simulink model "Cont_fullstate"  (R2020a)
settings: Solver=ode45  StartTime=0.0  StopTime=20  RelTol=1e-5
values from neighbouring files (symbols this model uses):
  A = [   0       1               0           0 ... (first row only)    [main_code.m]
  Ad = sys_d.a    [main_code.m]
  B = [   0 ... (first row only)    [main_code.m]
  b = 0.5    [main_code.m]
  Bd = sys_d.b    [main_code.m]
  C = [1   0   0   0 ... (first row only)    [main_code.m]
  Cd = sys_d.c    [main_code.m]
  Current_saturation = 2000    [main_code.m]
  D = [0 ... (first row only)    [main_code.m]
  Dd = sys_d.d    [main_code.m]
  g = 9.8    [main_code.m]
  I = (m*l^2)/3    (= 0.002646)    [main_code.m]
  K = lqr(A,B,Q,R)    [main_code.m]
  Kd = dlqr(Ad,Bd,Q,R)    [main_code.m]
  l = 0.21    [main_code.m]
  L = place(A',C',P)'    [main_code.m]
  Ld = place(Ad',Cd',Pd)'    [main_code.m]
  m = 0.18    [main_code.m]
  M = 0.195    [main_code.m]
  N_to_mAmp = 260    [main_code.m]
  Nc = 1/dcgain(sys_cl(1))    [main_code.m]
  Ndc = 1/dcgain(sys_d_cl(1))    [main_code.m]
  Ts = 1/100    (= 0.01)    [main_code.m]
  X0 = [0 0 pi 0.1]'    [main_code.m]
undefined symbols (not defined in the file or in its folder): X, Y, Z
libraries: sm_lib x8, nesl_utility x6
settings Model: Creator=imkis  LastModifiedBy=imkis
settings SolverCC: AlgebraicLoopSolver=LineSearch

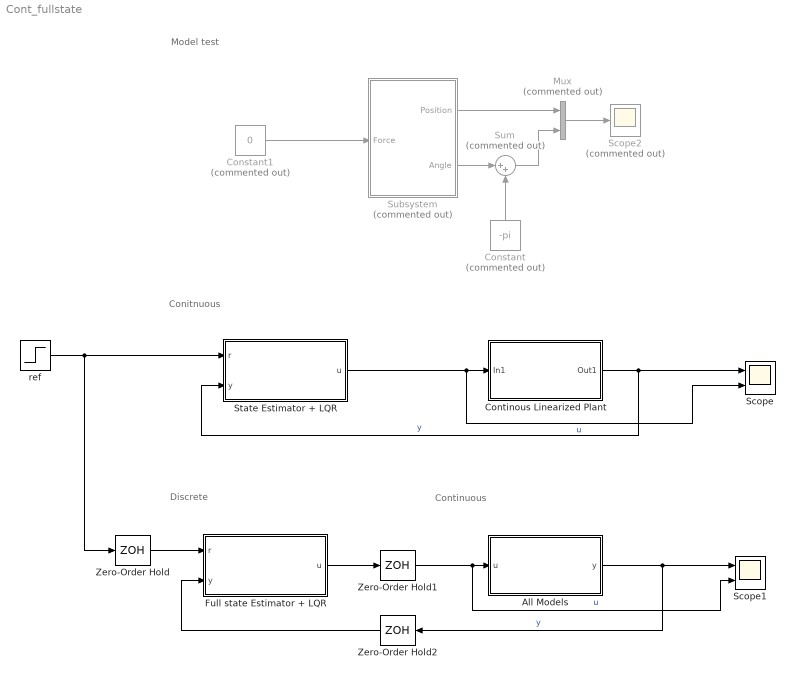
== system Cont_fullstate ==
  note: Model test
  note: Conitnuous
  note: Continuous
  note: Discrete
  All Models : Subsystem
  Constant : Constant  Commented=on  Value=-pi
  Constant1 : Constant  Commented=on  Value=0
  Continous Linearized Plant : Subsystem
  "Full state Estimator + LQR " : Subsystem
  Mux : Mux  Commented=on  Inputs=2
  Scope : Scope  NumInputPorts=2
  Scope1 : Scope  NumInputPorts=2
  Scope2 : Scope  Commented=on
  "State Estimator + LQR " : Subsystem
  Subsystem : Subsystem  Commented=on
  Sum : Sum  Commented=on  Inputs=|++
  Zero-Order Hold : ZeroOrderHold  SampleTime=Ts
  Zero-Order Hold1 : ZeroOrderHold  SampleTime=Ts
  Zero-Order Hold2 : ZeroOrderHold  SampleTime=Ts
  ref : Step  After=0.1  SampleTime=0
  wires:
  Continous Linearized Plant/1(Out1) -> Scope/1, "State Estimator + LQR "/2(y)  "y"
  "State Estimator + LQR "/1(u) -> Scope/2, Continous Linearized Plant/1(In1)  "u"
  ref/1 -> Zero-Order Hold/1, "State Estimator + LQR "/1(r)
  Zero-Order Hold/1 -> "Full state Estimator + LQR "/1(r)
  "Full state Estimator + LQR "/1(u) -> Zero-Order Hold1/1
  All Models/1(y) -> Scope1/1, Zero-Order Hold2/1  "y"
  Zero-Order Hold1/1 -> Scope1/2, All Models/1(u)  "u"
  Zero-Order Hold2/1 -> "Full state Estimator + LQR "/2(y)
  Subsystem/2(Angle) -> Sum/1
  Mux/1 -> Scope2/1
  Constant1/1 -> Subsystem/1(Force)
  Sum/1 -> Mux/2
  Subsystem/1(Position) -> Mux/1
  Constant/1 -> Sum/2

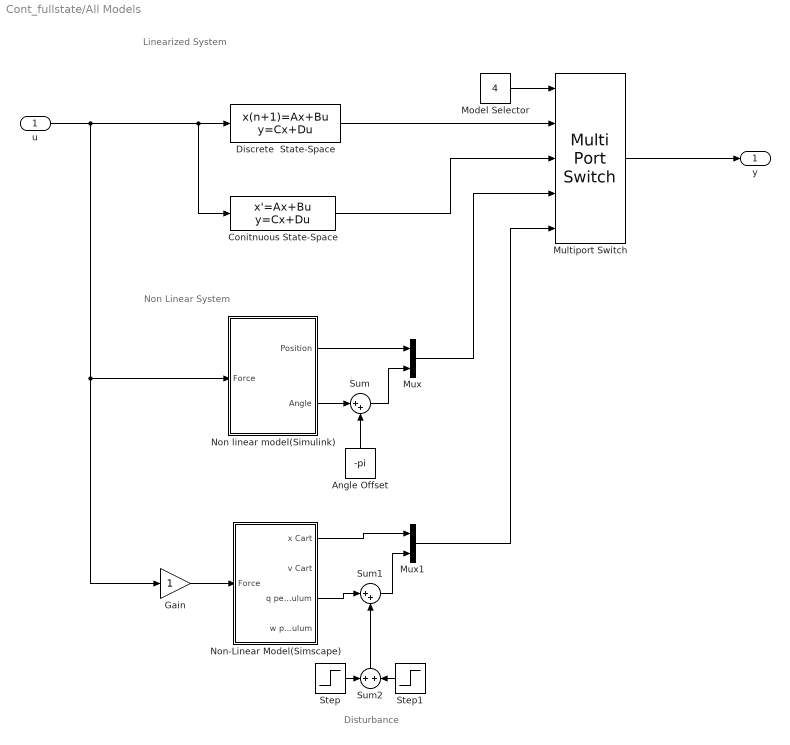
== system Cont_fullstate/All Models ==
  note: Disturbance
  note: Non Linear System
  note: Linearized System
  u : Inport
  Angle Offset : Constant  Value=-pi
  Conitnuous State-Space : StateSpace  A=A  B=B  C=C  D=D  InitialCondition=X0
  Discrete  State-Space : DiscreteStateSpace  A=Ad  B=Bd  C=Cd  D=Dd  InitialCondition=X0  SampleTime=Ts
  Gain : Gain
  Model Selector : Constant  Value=4
  Multiport Switch : MultiPortSwitch  Inputs=4
  Mux : Mux  Inputs=2
  Mux1 : Mux  Inputs=2
  "Non linear model(Simulink) " : Subsystem
  Non-Linear Model(Simscape) : Subsystem
  Step : Step  Time=5  After=0.1  SampleTime=0
  Step1 : Step  Time=5.05  After=-0.1  SampleTime=0
  Sum : Sum  Inputs=|++
  Sum1 : Sum  Inputs=|++
  Sum2 : Sum  Inputs=+|+
  y : Outport
  wires:
  Discrete  State-Space/1 -> Multiport Switch/2
  Conitnuous State-Space/1 -> Multiport Switch/3
  Multiport Switch/1 -> y/1
  "Non linear model(Simulink) "/2(Angle) -> Sum/1
  u/1 -> Conitnuous State-Space/1, Discrete  State-Space/1, "Non linear model(Simulink) "/1(Force), Gain/1
  Sum/1 -> Mux/2
  "Non linear model(Simulink) "/1(Position) -> Mux/1
  Angle Offset/1 -> Sum/2
  Sum1/1 -> Mux1/2
  Non-Linear Model(Simscape)/3(q pendulum) -> Sum1/1
  Non-Linear Model(Simscape)/1(x Cart) -> Mux1/1
  Mux1/1 -> Multiport Switch/5
  Mux/1 -> Multiport Switch/4
  Model Selector/1 -> Multiport Switch/1
  Gain/1 -> Non-Linear Model(Simscape)/1(Force)
  Step/1 -> Sum2/1
  Step1/1 -> Sum2/2
  Sum2/1 -> Sum1/2

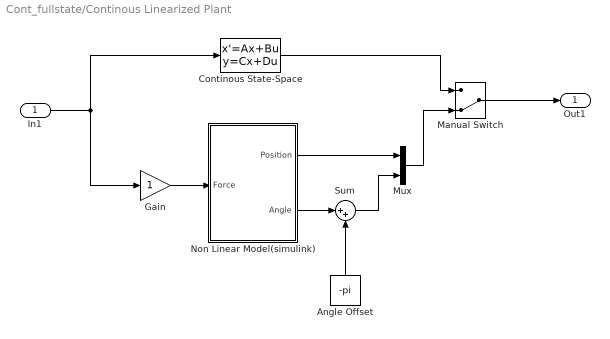
== system Cont_fullstate/Continous Linearized Plant ==
  In1 : Inport
  Angle Offset : Constant  Value=-pi
  Continous State-Space : StateSpace  A=A  B=B  C=C  D=D  InitialCondition=X0
  Gain : Gain
  Manual Switch : ManualSwitch  CurrentSetting=0
  Mux : Mux  Inputs=2
  Non Linear Model(simulink) : Subsystem
  Sum : Sum  Inputs=|++
  Out1 : Outport
  wires:
  Continous State-Space/1 -> Manual Switch/1
  Gain/1 -> Non Linear Model(simulink)/1(Force)
  Mux/1 -> Manual Switch/2
  Manual Switch/1 -> Out1/1
  Non Linear Model(simulink)/2(Angle) -> Sum/1
  Sum/1 -> Mux/2
  Non Linear Model(simulink)/1(Position) -> Mux/1
  Angle Offset/1 -> Sum/2
  In1/1 -> Continous State-Space/1, Gain/1

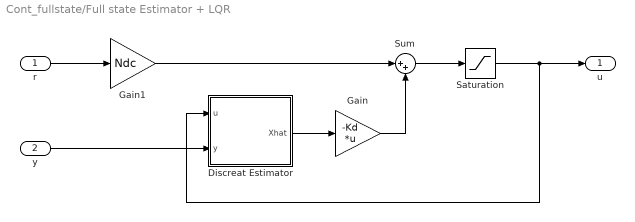
== system Cont_fullstate/Full state Estimator + LQR  ==
  r : Inport
  y : Inport  Port=2
  Discreat Estimator : Subsystem
  Gain : Gain  Gain=-Kd  Multiplication=Matrix(K*u)
  Gain1 : Gain  Gain=Ndc
  Saturation : Saturate  UpperLimit=Current_saturation/N_to_mAmp  LowerLimit=-Current_saturation/N_to_mAmp
  Sum : Sum  Inputs=|++
  u : Outport
  wires:
  Gain1/1 -> Sum/1
  Sum/1 -> Saturation/1
  y/1 -> Discreat Estimator/2(y)
  Discreat Estimator/1(Xhat) -> Gain/1
  Gain/1 -> Sum/2
  r/1 -> Gain1/1
  Saturation/1 -> u/1, Discreat Estimator/1(u)

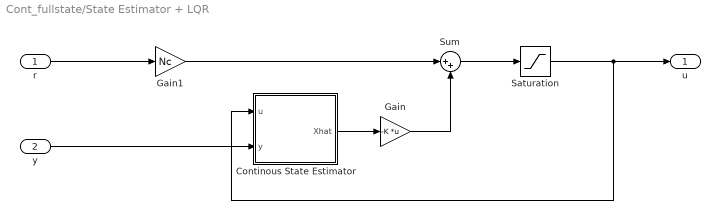
== system Cont_fullstate/State Estimator + LQR  ==
  r : Inport
  y : Inport  Port=2
  Continous State Estimator : Subsystem
  Gain : Gain  Gain=-K  Multiplication=Matrix(K*u)
  Gain1 : Gain  Gain=Nc
  Saturation : Saturate  UpperLimit=8  LowerLimit=-8
  Sum : Sum  Inputs=|++
  u : Outport
  wires:
  Gain1/1 -> Sum/1
  Sum/1 -> Saturation/1
  y/1 -> Continous State Estimator/2(y)
  Continous State Estimator/1(Xhat) -> Gain/1
  Gain/1 -> Sum/2
  r/1 -> Gain1/1
  Saturation/1 -> Continous State Estimator/1(u), u/1

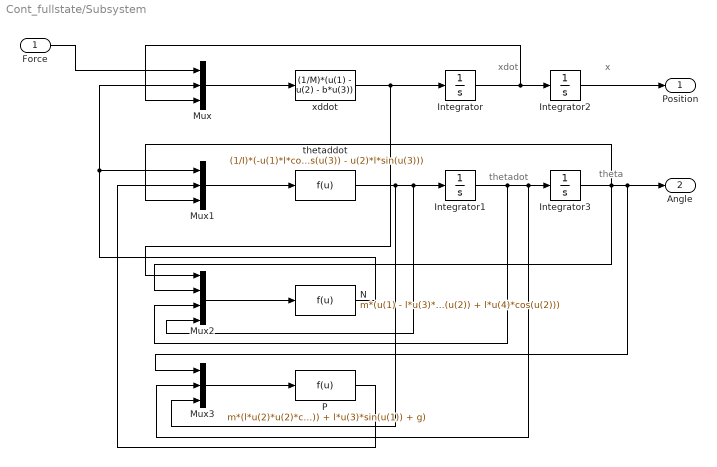
== system Cont_fullstate/Subsystem ==
  note: theta
  note: x
  note: thetadot
  note: xdot
  Force : Inport
  Integrator : Integrator  InitialCondition=X0(2)  ContinuousStateAttributes='xdot'
  Integrator1 : Integrator  InitialCondition=X0(4)  ContinuousStateAttributes='thetadot'
  Integrator2 : Integrator  InitialCondition=X0(1)  ContinuousStateAttributes='x'
  Integrator3 : Integrator  InitialCondition=X0(3)  ContinuousStateAttributes='theta'
  Mux : Mux  Inputs=3
  Mux1 : Mux  Inputs=3
  Mux2 : Mux
  Mux3 : Mux  Inputs=3
  N : Fcn  Expr=m*(u(1) - l*u(3)*u(3)*sin(u(2)) + l*u(4)*cos(u(2)))
  P : Fcn  Expr=m*(l*u(2)*u(2)*cos(u(1)) + l*u(3)*sin(u(1)) + g)
  thetaddot : Fcn  Expr=(1/I)*(-u(1)*l*cos(u(3)) - u(2)*l*sin(u(3)))
  xddot : Fcn  Expr=(1/M)*(u(1) - u(2) - b*u(3))
  Position : Outport
  Angle : Outport  Port=2
  wires:
  Force/1 -> Mux/1
  Mux2/1 -> N/1
  Mux/1 -> xddot/1
  P/1 -> Mux1/2
  Mux3/1 -> P/1
  N/1 -> Mux1/1, Mux/2
  Mux1/1 -> thetaddot/1
  xddot/1 -> Mux2/1, Integrator/1
  Integrator2/1 -> Position/1
  thetaddot/1 -> Mux3/3, Mux2/4, Integrator1/1
  Integrator/1 -> Mux/3, Integrator2/1
  Integrator1/1 -> Mux2/3, Mux3/2, Integrator3/1
  Integrator3/1 -> Mux2/2, Mux1/3, Angle/1, Mux3/1

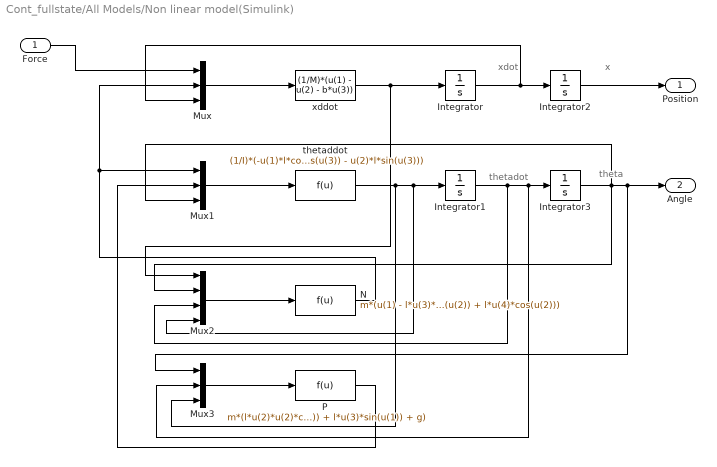
== system Cont_fullstate/All Models/Non linear model(Simulink)  ==
  note: theta
  note: x
  note: thetadot
  note: xdot
  Force : Inport
  Integrator : Integrator  ContinuousStateAttributes='xdot'
  Integrator1 : Integrator  ContinuousStateAttributes='thetadot'
  Integrator2 : Integrator  ContinuousStateAttributes='x'
  Integrator3 : Integrator  InitialCondition=pi  ContinuousStateAttributes='theta'
  Mux : Mux  Inputs=3
  Mux1 : Mux  Inputs=3
  Mux2 : Mux
  Mux3 : Mux  Inputs=3
  N : Fcn  Expr=m*(u(1) - l*u(3)*u(3)*sin(u(2)) + l*u(4)*cos(u(2)))
  P : Fcn  Expr=m*(l*u(2)*u(2)*cos(u(1)) + l*u(3)*sin(u(1)) + g)
  thetaddot : Fcn  Expr=(1/I)*(-u(1)*l*cos(u(3)) - u(2)*l*sin(u(3)))
  xddot : Fcn  Expr=(1/M)*(u(1) - u(2) - b*u(3))
  Position : Outport
  Angle : Outport  Port=2
  wires:
  Force/1 -> Mux/1
  Mux2/1 -> N/1
  Mux/1 -> xddot/1
  P/1 -> Mux1/2
  Mux3/1 -> P/1
  N/1 -> Mux1/1, Mux/2
  Mux1/1 -> thetaddot/1
  xddot/1 -> Mux2/1, Integrator/1
  Integrator2/1 -> Position/1
  thetaddot/1 -> Mux3/3, Mux2/4, Integrator1/1
  Integrator/1 -> Mux/3, Integrator2/1
  Integrator1/1 -> Mux2/3, Mux3/2, Integrator3/1
  Integrator3/1 -> Mux2/2, Mux1/3, Angle/1, Mux3/1

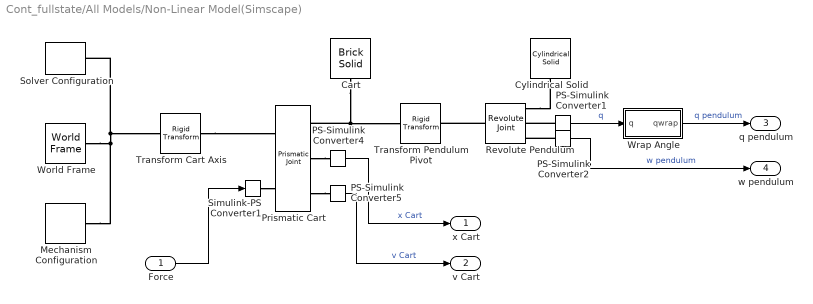
== system Cont_fullstate/All Models/Non-Linear Model(Simscape) ==
  Force : Inport
  Cart : sm_lib/Body Elements/Brick Solid  GraphicAmbientColor=[0.15 0.15 0.15 1.0]  BasedOnType=Density  BrickDimensions=[0.05 0.05 0.05]  BrickDimensionUnits=m  CenterOfMass=[0 0 0]  CenterOfMassUnits=m  GraphicDiffuseColor=[0.8 0.45 0]  Density=1000  DensityUnits=kg/m^3  DoExposeReferenceFrame=on  GraphicEmissiveColor=[0.0 0.0 0.0 1.0]  ExportEntireGeometry=off  SerializedFrames=<Frames/>  MarkerShape=Sphere  MarkerSize=10  GraphicType=FromGeometry  InertiaType=PointMass  Mass=M  MassUnits=kg  MomentsOfInertia=[1 1 1]  MomentsOfInertiaUnits=kg*m^2  GraphicOpacity=1.0  ProductsOfInertia=[0 0 0]  ProductsOfInertiaUnits=kg*m^2  GraphicShininess=75  GraphicSpecularColor=[0.5 0.5 0.5 1.0]  GraphicVisPropType=SimpleVisualProperties
  Cylindrical Solid : sm_lib/Body Elements/Cylindrical Solid  GraphicAmbientColor=[0.15 0.15 0.15 1.0]  BasedOnType=Mass  CenterOfMass=[0 0 0]  CenterOfMassUnits=m  GraphicDiffuseColor=[0.5 0.5 0.5]  CylinderLength=l*2  CylinderLengthUnits=m  CylinderRadius=0.004  CylinderRadiusUnits=m  Density=1000  DensityUnits=kg/m^3  DoExposeReferenceFrame=off  GraphicEmissiveColor=[0.0 0.0 0.0 1.0]  ExportEntireGeometry=off  SerializedFrames=<Frames><Frame><Id>Frame1</Id><Value><Name>B</Name><Origin><Source>GeometricFeature</Source><FeatureName>bottom curve</FeatureName></Origin><PrimaryAxis><DefinedDirection>-X</DefinedDirection><Source>ReferenceFrame</Source><SourceDirection>+Z</SourceDirection><FeatureName></FeatureName></PrimaryAxis><SecondaryAxis><DefinedDirection>+Y</DefinedDirection><Source>ReferenceFrame</Source><SourceDirection>+X</SourceDirection><FeatureName></FeatureName></SecondaryAxis></Value></Frame></Frames>  MarkerShape=Sphere  MarkerSize=10  GraphicType=FromGeometry  InertiaType=CalculateFromGeometry  Mass=m  MassUnits=kg  MomentsOfInertia=[1 1 1]  MomentsOfInertiaUnits=kg*m^2  GraphicOpacity=1.0  ProductsOfInertia=[0 0 0]  ProductsOfInertiaUnits=kg*m^2  GraphicShininess=75  GraphicSpecularColor=[0.5 0.5 0.5 1.0]  GraphicVisPropType=SimpleVisualProperties
  Mechanism Configuration : sm_lib/Utilities/Mechanism Configuration  UniformGravity=Constant  GravityVector=[0 0 -9.80665]  GravityUnits=m/s^2  LinearizationDelta=0.001
  PS-Simulink Converter1 : nesl_utility/PS-Simulink Converter  PhysicalDomain=network_engine_domain  SubClassName=ps_output  LeftPortType=input  RightPortType=output  PseudoPeriodic=off  Frequencies=[]  Unit=rad  AffineConversion=off
  PS-Simulink Converter2 : nesl_utility/PS-Simulink Converter  PhysicalDomain=network_engine_domain  SubClassName=ps_output  LeftPortType=input  RightPortType=output  PseudoPeriodic=off  Frequencies=[]  Unit=rad/s  AffineConversion=off
  PS-Simulink Converter4 : nesl_utility/PS-Simulink Converter  PhysicalDomain=network_engine_domain  SubClassName=ps_output  LeftPortType=input  RightPortType=output  PseudoPeriodic=off  Frequencies=[]  Unit=m  AffineConversion=off
  PS-Simulink Converter5 : nesl_utility/PS-Simulink Converter  PhysicalDomain=network_engine_domain  SubClassName=ps_output  LeftPortType=input  RightPortType=output  PseudoPeriodic=off  Frequencies=[]  Unit=m/s  AffineConversion=off
  Prismatic Cart : sm_lib/Joints/Prismatic Joint  JointMode=Normal  SenseConstraintForce=off  SenseConstraintForceX=off  SenseConstraintForceY=off  SenseConstraintForceZ=off  SenseConstraintTorque=off  SenseConstraintTorqueX=off  SenseConstraintTorqueY=off  SenseConstraintTorqueZ=off  SenseTotalForce=off  SenseTotalForceX=off  SenseTotalForceY=off  SenseTotalForceZ=off  SenseTotalTorque=off  SenseTotalTorqueX=off  SenseTotalTorqueY=off  SenseTotalTorqueZ=off  CompositeWrenchDir=FollowerOnBase  CompositeWrenchFrame=BaseFrame  EquilibriumPosition=0  EquilibriumPositionUnits=m  SpringStiffness=0  SpringStiffnessUnits=N/m  DampingCoefficient=b  DampingCoefficientUnits=N/(m/s)  TorqueActuationMode=InputTorque  MotionActuationMode=ComputedMotion  SensePosition=on  SenseVelocity=on  SenseAcceleration=off  SenseTorqueForce=off  SenseLowerLimitTorqueForce=off  SenseUpperLimitTorqueForce=off  LowerLimitSpecify=on  LowerLimitBound=-0.2  LowerLimitBoundUnits=m  LowerLimitStiffness=1e6  LowerLimitStiffnessUnits=N/m  LowerLimitDamping=1e3  LowerLimitDampingUnits=N/(m/s)  LowerLimitTransitionRegionWidth=1e-4  LowerLimitTransitionRegionWidthUnits=m  UpperLimitSpecify=on  UpperLimitBound=0.2  UpperLimitBoundUnits=m  UpperLimitStiffness=1e6  UpperLimitStiffnessUnits=N/m  UpperLimitDamping=1e3  UpperLimitDampingUnits=N/(m/s)  UpperLimitTransitionRegionWidth=1e-4  UpperLimitTransitionRegionWidthUnits=m  PositionTargetSpecify=off  PositionTargetPriority=High  PositionTargetValue=0  PositionTargetValueUnits=m  VelocityTargetSpecify=off  VelocityTargetPriority=High  VelocityTargetValue=0  VelocityTargetValueUnits=m/s
  Revolute Pendulum : sm_lib/Joints/Revolute Joint  JointMode=Normal  SenseConstraintForce=off  SenseConstraintForceX=off  SenseConstraintForceY=off  SenseConstraintForceZ=off  SenseConstraintTorque=off  SenseConstraintTorqueX=off  SenseConstraintTorqueY=off  SenseConstraintTorqueZ=off  SenseTotalForce=off  SenseTotalForceX=off  SenseTotalForceY=off  SenseTotalForceZ=off  SenseTotalTorque=off  SenseTotalTorqueX=off  SenseTotalTorqueY=off  SenseTotalTorqueZ=off  CompositeWrenchDir=FollowerOnBase  CompositeWrenchFrame=BaseFrame  EquilibriumPosition=0  EquilibriumPositionUnits=deg  SpringStiffness=0  SpringStiffnessUnits=N*m/deg  DampingCoefficient=0  DampingCoefficientUnits=N*m/(deg/s)  TorqueActuationMode=NoTorque  MotionActuationMode=ComputedMotion  SensePosition=on  SenseVelocity=on  SenseAcceleration=off  SenseTorqueForce=off  SenseLowerLimitTorqueForce=off  SenseUpperLimitTorqueForce=off  LowerLimitSpecify=off  LowerLimitBound=-90  LowerLimitBoundUnits=deg  LowerLimitStiffness=1e4  LowerLimitStiffnessUnits=N*m/deg  LowerLimitDamping=10  LowerLimitDampingUnits=N*m/(deg/s)  LowerLimitTransitionRegionWidth=0.1  LowerLimitTransitionRegionWidthUnits=deg  UpperLimitSpecify=off  UpperLimitBound=90  UpperLimitBoundUnits=deg  UpperLimitStiffness=1e4  UpperLimitStiffnessUnits=N*m/deg  UpperLimitDamping=10  UpperLimitDampingUnits=N*m/(deg/s)  UpperLimitTransitionRegionWidth=0.1  UpperLimitTransitionRegionWidthUnits=deg  PositionTargetSpecify=off  PositionTargetPriority=High  PositionTargetValue=0  PositionTargetValueUnits=deg  VelocityTargetSpecify=off  VelocityTargetPriority=High  VelocityTargetValue=0  VelocityTargetValueUnits=deg/s
  Simulink-PS Converter1 : nesl_utility/Simulink-PS Converter  PhysicalDomain=network_engine_domain  SubClassName=ps_input  LeftPortType=input  RightPortType=output  PseudoPeriodic=off  Frequencies=[]  NoiseDistribution=none  NoiseParameters=[]  Unit=N  AffineConversion=off  FilteringAndDerivatives=zero  SimscapeFilterOrder=1  InputFilterTimeConstant=.001  UdotUserProvided=1
  Solver Configuration : nesl_utility/Solver Configuration  PhysicalDomain=network_engine_domain  SubClassName=solver  LeftPortType=input  RightPortType=generic  Tones=[]  Harmonics=[]  SimulateNoise=off  Profile=off  UseLocalSampling=off  EnableSwitchedLinearOptims=on  FrequencyDomain=off  UseCCode=off  RelTol=0.001  AbsTol=1e-06  MinStep=1e-09  ToWorkspace=off  RevertToSquareIcSolve=off  NumHomotopyIterations=100  PhasorMode=off  PhasorModeNumHarmonics=1  DoDC=off  ResidualTolerance=1e-09  UseLocalSolver=off  LocalSolverChoice=NE_BACKWARD_EULER_ADVANCER  LocalSolverSampleTime=0.001  DoFixedCost=off  MaxNonlinIter=3  MaxModeIter=2  LinearAlgebra=Sparse  EquationFormulation=NE_TIME_EF  DelaysMemoryBudget=1024  AutomaticFiltering=on  FilteringTimeConstant=0.001  PartitionStorageMethod=AS_NEEDED  PartitionMemoryBudget=1024  PartitionMethod=FAST
  Transform Cart Axis : sm_lib/Frames and Transforms/Rigid Transform  TranslationMethod=None  TranslationStandardOffset=0  TranslationLengthUnit=m  TranslationStandardAxis=+Z  TranslationCartesianOffset=[0 0 0]  TranslationROffset=0  TranslationROffsetUnits=m  TranslationZOffset=0  TranslationZOffsetUnits=m  TranslationThetaOffset=0  TranslationThetaOffsetUnits=deg  RotationMethod=StandardAxis  RotationAngleUnits=deg  RotationStandardAxis=+Y  RotationAngle=90  RotationArbitraryAxis=[0 0 1]  FollAlignAxisA=+X  BaseAlignAxisA=+Y  FollAlignAxisB=+Y  BaseAlignAxisB=+Z  RotationSequenceAxes=FollowerAxes  RotationSequence=XYX  RotationSequenceAngles=[0 0 0]  RotationSequenceAnglesUnits=deg  RotationMatrix=[1 0 0; 0 1 0; 0 0 1]
  Transform Pendulum Pivot : sm_lib/Frames and Transforms/Rigid Transform  TranslationMethod=None  TranslationStandardOffset=0.025  TranslationLengthUnit=m  TranslationStandardAxis=-X  TranslationCartesianOffset=[0 0 0]  TranslationROffset=0  TranslationROffsetUnits=m  TranslationZOffset=0  TranslationZOffsetUnits=m  TranslationThetaOffset=0  TranslationThetaOffsetUnits=deg  RotationMethod=StandardAxis  RotationAngleUnits=deg  RotationStandardAxis=+X  RotationAngle=90  RotationArbitraryAxis=[0 0 1]  FollAlignAxisA=+X  BaseAlignAxisA=+Y  FollAlignAxisB=+Y  BaseAlignAxisB=+Z  RotationSequenceAxes=FollowerAxes  RotationSequence=XYX  RotationSequenceAngles=[0 0 0]  RotationSequenceAnglesUnits=deg  RotationMatrix=[1 0 0; 0 1 0; 0 0 1]
  World Frame : sm_lib/Frames and Transforms/World Frame
  Wrap Angle : Subsystem
  x Cart : Outport  VectorParamsAs1DForOutWhenUnconnected=off
  v Cart : Outport  Port=2  VectorParamsAs1DForOutWhenUnconnected=off
  q pendulum : Outport  Port=3  VectorParamsAs1DForOutWhenUnconnected=off
  w pendulum : Outport  Port=4  VectorParamsAs1DForOutWhenUnconnected=off
  wires:
  PS-Simulink Converter1/1 -> Wrap Angle/1(q)  "q"
  Force/1 -> Simulink-PS Converter1/1
  PS-Simulink Converter4/1 -> x Cart/1  "x Cart"
  PS-Simulink Converter5/1 -> v Cart/1  "v Cart"
  PS-Simulink Converter2/1 -> w pendulum/1  "w pendulum"
  Wrap Angle/1(qwrap) -> q pendulum/1  "q pendulum"
  connections:
  Revolute Pendulum/LConn1 -- Transform Pendulum Pivot/RConn1
  Prismatic Cart/RConn2 -- PS-Simulink Converter4/LConn1
  PS-Simulink Converter1/LConn1 -- Revolute Pendulum/RConn2
  Revolute Pendulum/RConn1 -- Cylindrical Solid/LConn1
  Cart/RConn1 -- Prismatic Cart/RConn1 -- Transform Pendulum Pivot/LConn1
  Prismatic Cart/RConn3 -- PS-Simulink Converter5/LConn1
  PS-Simulink Converter2/LConn1 -- Revolute Pendulum/RConn3
  Simulink-PS Converter1/RConn1 -- Prismatic Cart/LConn2
  Solver Configuration/RConn1 -- Transform Cart Axis/LConn1 -- Mechanism Configuration/RConn1 -- World Frame/RConn1
  Transform Cart Axis/RConn1 -- Prismatic Cart/LConn1

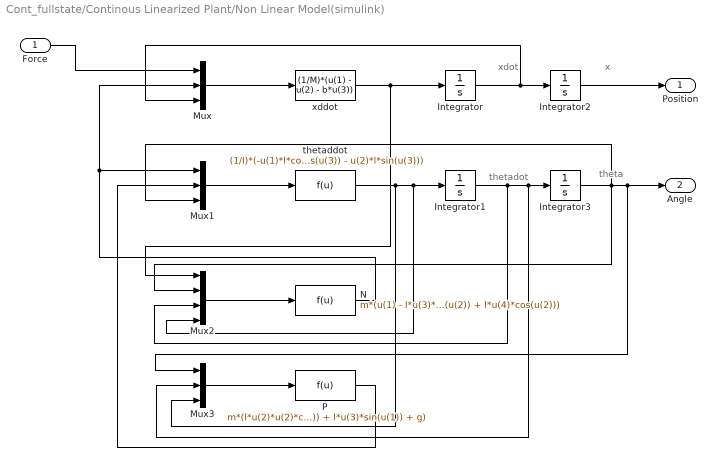
== system Cont_fullstate/Continous Linearized Plant/Non Linear Model(simulink) ==
  note: theta
  note: x
  note: thetadot
  note: xdot
  Force : Inport
  Integrator : Integrator  ContinuousStateAttributes='xdot'
  Integrator1 : Integrator  ContinuousStateAttributes='thetadot'
  Integrator2 : Integrator  ContinuousStateAttributes='x'
  Integrator3 : Integrator  InitialCondition=pi  ContinuousStateAttributes='theta'
  Mux : Mux  Inputs=3
  Mux1 : Mux  Inputs=3
  Mux2 : Mux
  Mux3 : Mux  Inputs=3
  N : Fcn  Expr=m*(u(1) - l*u(3)*u(3)*sin(u(2)) + l*u(4)*cos(u(2)))
  P : Fcn  Expr=m*(l*u(2)*u(2)*cos(u(1)) + l*u(3)*sin(u(1)) + g)
  thetaddot : Fcn  Expr=(1/I)*(-u(1)*l*cos(u(3)) - u(2)*l*sin(u(3)))
  xddot : Fcn  Expr=(1/M)*(u(1) - u(2) - b*u(3))
  Position : Outport
  Angle : Outport  Port=2
  wires:
  Force/1 -> Mux/1
  Mux2/1 -> N/1
  Mux/1 -> xddot/1
  P/1 -> Mux1/2
  Mux3/1 -> P/1
  N/1 -> Mux1/1, Mux/2
  Mux1/1 -> thetaddot/1
  xddot/1 -> Mux2/1, Integrator/1
  Integrator2/1 -> Position/1
  thetaddot/1 -> Mux3/3, Mux2/4, Integrator1/1
  Integrator/1 -> Mux/3, Integrator2/1
  Integrator1/1 -> Mux2/3, Mux3/2, Integrator3/1
  Integrator3/1 -> Mux2/2, Mux1/3, Angle/1, Mux3/1

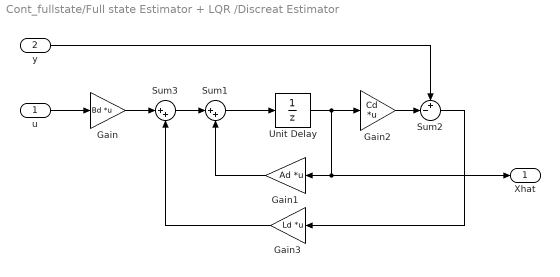
== system Cont_fullstate/Full state Estimator + LQR /Discreat Estimator ==
  u : Inport
  y : Inport  Port=2
  Gain : Gain  Gain=Bd  Multiplication=Matrix(K*u)
  Gain1 : Gain  Gain=Ad  Multiplication=Matrix(K*u)
  Gain2 : Gain  Gain=Cd  Multiplication=Matrix(K*u)
  Gain3 : Gain  Gain=Ld  Multiplication=Matrix(K*u)
  Sum1 : Sum  Inputs=|++
  Sum2 : Sum  Inputs=+-|
  Sum3 : Sum  Inputs=|++
  Unit Delay : UnitDelay  SampleTime=Ts  HasFrameUpgradeWarning=on
  Xhat : Outport
  wires:
  u/1 -> Gain/1
  y/1 -> Sum2/1
  Sum2/1 -> Gain3/1
  Sum1/1 -> Unit Delay/1
  Unit Delay/1 -> Xhat/1, Gain1/1, Gain2/1
  Gain2/1 -> Sum2/2
  Gain1/1 -> Sum1/2
  Gain3/1 -> Sum3/2
  Sum3/1 -> Sum1/1
  Gain/1 -> Sum3/1

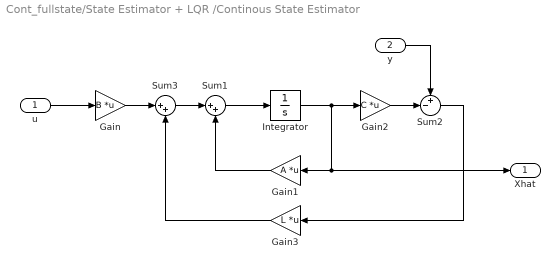
== system Cont_fullstate/State Estimator + LQR /Continous State Estimator ==
  u : Inport
  y : Inport  Port=2
  Gain : Gain  Gain=B  Multiplication=Matrix(K*u)
  Gain1 : Gain  Gain=A  Multiplication=Matrix(K*u)
  Gain2 : Gain  Gain=C  Multiplication=Matrix(K*u)
  Gain3 : Gain  Gain=L  Multiplication=Matrix(K*u)
  Integrator : Integrator
  Sum1 : Sum  Inputs=|++
  Sum2 : Sum  Inputs=+-|
  Sum3 : Sum  Inputs=|++
  Xhat : Outport
  wires:
  u/1 -> Gain/1
  y/1 -> Sum2/1
  Sum2/1 -> Gain3/1
  Sum1/1 -> Integrator/1
  Integrator/1 -> Xhat/1, Gain1/1, Gain2/1
  Gain2/1 -> Sum2/2
  Gain1/1 -> Sum1/2
  Gain3/1 -> Sum3/2
  Sum3/1 -> Sum1/1
  Gain/1 -> Sum3/1

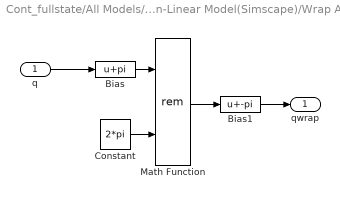
== system Cont_fullstate/All Models/Non-Linear Model(Simscape)/Wrap Angle ==
  q : Inport
  Bias : Bias  Bias=pi
  Bias1 : Bias  Bias=-pi
  Constant : Constant  Value=2*pi
  Math Function : Math  Operator=rem  SignedPower=on  SaturateOnIntegerOverflow=on
  qwrap : Outport  VectorParamsAs1DForOutWhenUnconnected=off
  wires:
  q/1 -> Bias/1
  Constant/1 -> Math Function/2
  Math Function/1 -> Bias1/1
  Bias/1 -> Math Function/1
  Bias1/1 -> qwrap/1
